simulink model "DC_Motor"  (R2018a)
settings: Solver=VariableStepAuto  StartTime=0.0  StopTime=10  RelTol=1e-3
libraries: simulink x1
settings Model: Creator=Jayef  LastModifiedBy=Jayef

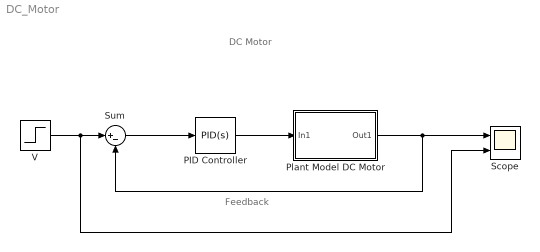
== system DC_Motor ==
  note: DC Motor
  note: Feedback
  PID Controller : simulink/Continuous/PID Controller  Controller=PID  TimeDomain=Continuous-time  SampleTime=-1  IntegratorMethod=Forward Euler  FilterMethod=Forward Euler  Form=Parallel  UseFilter=on  ControllerParametersSource=internal  P=1.33985893874321  I=5.65629390629391  D=0.0252736741105271  N=5544.98326466803  InitialConditionSource=internal  InitialConditionForIntegrator=0  InitialConditionForFilter=0  ExternalReset=none  LimitOutput=off  UpperSaturationLimit=inf  LowerSaturationLimit=-inf  LinearizeAsGain=on  AntiWindupMode=none  Kb=1  TrackingMode=off  Kt=1  PParamMin=[]  PParamMax=[]  IParamMin=[]  IParamMax=[]  DParamMin=[]  DParamMax=[]  NParamMin=[]  NParamMax=[]  KbParamMin=[]  KbParamMax=[]  KtParamMin=[]  KtParamMax=[]  POutMin=[]  POutMax=[]  IOutMin=[]  IOutMax=[]  DOutMin=[]  DOutMax=[]  NOutMin=[]  NOutMax=[]  KbOutMin=[]  KbOutMax=[]  KtOutMin=[]  KtOutMax=[]  IntegratorOutMin=[]  IntegratorOutMax=[]  FilterOutMin=[]  FilterOutMax=[]  SumOutMin=[]  SumOutMax=[]  SumI1OutMin=[]  SumI1OutMax=[]  SumI2OutMin=[]  SumI2OutMax=[]  SumI3OutMin=[]  SumI3OutMax=[]  SumDOutMin=[]  SumDOutMax=[]  SaturationOutMin=[]  SaturationOutMax=[]  IntegratorContinuousStateAttributes=''  IntegratorStateMustResolveToSignalObject=off  IntegratorRTWStateStorageClass=Auto  FilterContinuousStateAttributes=''  FilterStateMustResolveToSignalObject=off  FilterRTWStateStorageClass=Auto  DifferentiatorICPrevScaledInput=0  DifferentiatorOutMin=[]  DifferentiatorOutMax=[]  FilterDiffOutCoefMin=[]  FilterDiffOutCoefMax=[]  SumDenOutMin=[]  SumDenOutMax=[]  SumNumOutMin=[]  SumNumOutMax=[]  ReciprocalOutMin=[]  ReciprocalOutMax=[]  DivideOutMin=[]  DivideOutMax=[]  TunerSelectOption=Transfer Function Based (PID Tuner App)
  Plant Model DC Motor : Subsystem
  Scope : Scope  NumInputPorts=2
  Sum : Sum  Inputs=|+-
  V : Step  SampleTime=0
  wires:
  PID Controller/1 -> Plant Model DC Motor/1(In1)
  Sum/1 -> PID Controller/1
  V/1 -> Scope/2, Sum/1
  Plant Model DC Motor/1(Out1) -> Sum/2, Scope/1

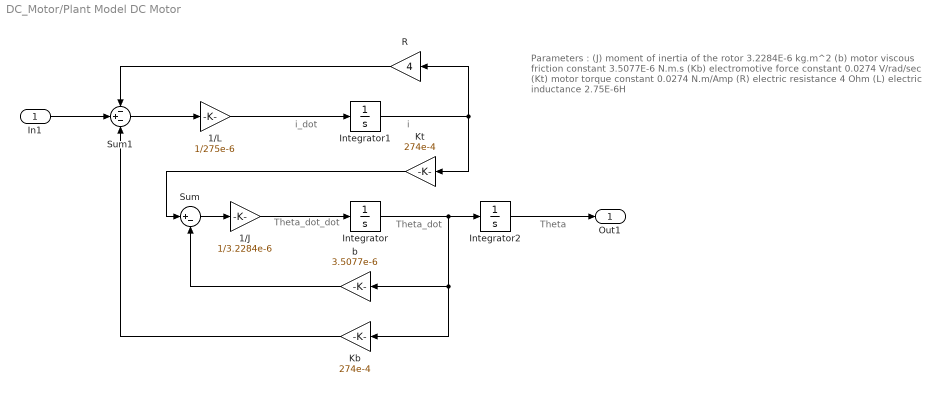
== system DC_Motor/Plant Model DC Motor ==
  note: i_dot
  note: i
  note: Theta
  note: Theta_dot_dot
  note: Theta_dot
  note: Parameters :
      | (J) moment of inertia of the rotor 3.2284E-6 kg.m^2
      | (b) motor viscous friction constant 3.5077E-6 N.m.s
      | (Kb) electromotive force constant 0.0274 V/rad/sec
      | (Kt) motor torque constant 0.0274 N.m/Amp
      | (R) electric resistance 4 Ohm
      | (L) electric inductance 2.75E-6H
  In1 : Inport
  1/J : Gain  Gain=1/3.2284e-6
  1/L : Gain  Gain=1/275e-6
  Integrator : Integrator
  Integrator1 : Integrator
  Integrator2 : Integrator
  Kb : Gain  Gain=274e-4
  Kt : Gain  Gain=274e-4
  R : Gain  Gain=4
  Sum : Sum  Inputs=|+-
  Sum1 : Sum  Inputs=-+-
  b : Gain  Gain=3.5077e-6
  Out1 : Outport
  wires:
  Sum1/1 -> 1/L/1
  Kb/1 -> Sum1/3
  1/L/1 -> Integrator1/1
  Integrator/1 -> Integrator2/1, Kb/1, b/1
  Integrator1/1 -> Kt/1, R/1
  R/1 -> Sum1/1
  1/J/1 -> Integrator/1
  b/1 -> Sum/2
  Kt/1 -> Sum/1
  Sum/1 -> 1/J/1
  In1/1 -> Sum1/2
  Integrator2/1 -> Out1/1
